simulink model "kyvadloMPC"  (R2018a)
settings: Solver=FixedStepAuto  StartTime=0.0  StopTime=10  FixedStep=Ts  MaxStep=0.01  RelTol=1e-3  EnableMultiTasking=on
PreLoadFcn:
  | m1=0.4;        % Hmotnost vozika [kg]
  | m2=0.08;      % Hmotnost kyvadla [kg]
  | l=0.2;            % Vzdialenost taziska od osi rotacie [m]
  | g=9.81;         % Tiazove zrychlenie [m/s2]
  | b=0.1;           % Koeficient trenia [m/s]
StartFcn:
  | kyvadloOfflineMPC
values from neighbouring files (symbols this model uses):
  Ac = -1/tau    (= -0.0166666666667)    [integrator.m]    (also in obmedzenia.m = [Acu;Acx]; stavovyprikaz.m = [-0.313 56.7 0; -0.0139 -0.426 0; 0 56.7 0]; testrozsirenieintegrator.m)
  b0 = [b0u; b0x]    [obmedzenia.m]
  B0 = [zeros(2*p5*nu,nx); B0x]    [obmedzenia.m]
  G = G+N((i-1)*nx+1:i*nx,:)'*P*M((i-1)*nx+1:i*nx,:)    [ucelovafunkcia.m]
  H = (H+H')/2    [.m]    (also in MPCuzavretaslucka.m; inkrementalny.m; integrator.m; kombinovaneobmedzenia.m)
  Ts = 5    [integrator.m]    (also in kyvadloOfflineLQ.m = kyvadlo.Ts; kyvadloOfflineMPC.m = kyvadlo.Ts; kyvadloOfflineMPCaKF.m = kyvadlo.Ts; stavovyprikaz.m = 0.5)
  uh = 0.002    [.m]    (also in MPCjedenkrok.m = 0.01; MPCuzavretaslucka.m = 0.01; integrator.m = 10; kombinovaneobmedzenia.m = 0.005)
  ul = -uh    (= -0.01)    [MPCjedenkrok.m]    (also in MPCuzavretaslucka.m; integrator.m = 0; kyvadloOfflineLQ.m = -5; kyvadloOfflineMPC.m = -5)
  x1h = 0.5    [kyvadloOfflineLQ.m]    (also in kyvadloOfflineMPC.m; kyvadloOfflineMPCaKF.m)
  x1l = -x1h    (= -0.5)    [kyvadloOfflineLQ.m]    (also in kyvadloOfflineMPC.m; kyvadloOfflineMPCaKF.m)
settings Model: Creator=UAMAI-LENOVO  LastModifiedBy=Gergely
settings DataIOCC: LimitDataPoints=on  SaveFormat=Array
settings OptimizationCC: LifeSpan=inf
settings DebuggingCC: SFUnexpectedBacktrackingDiag=warning  SFNoUnconditionalDefaultTransitionDiag=warning  SFExecutionAtInitializationDiag=none
settings HardwareCC: ProdBitPerPointer=32  ProdBitPerSizeT=32  ProdBitPerPtrDiffT=32  ProdLargestAtomicFloat=None  ProdIntDivRoundTo=Undefined  ProdEndianess=Unspecified  ProdWordSize=32  ProdHWDeviceType=32-bit Generic
settings ModelReferenceCC: PropagateSignalLabelsOutOfModel=off
settings CodeAppCC: StateflowObjectComments=on
settings GRTTargetCC: TargetLangStandard=C89/C90 (ANSI)  GeneratePreprocessorConditionals=Disable all
settings ConfigComp: CovMetricSettings=dw  CovHtmlReporting=on  CovSaveCumulativeToWorkspaceVar=on  CovSaveSingleToWorkspaceVar=on  CovExternalEMLEnable=off

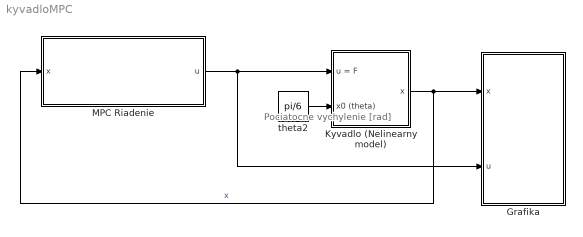
== system kyvadloMPC ==
  note: Pociatocne
      | vychylenie [rad]
  Grafika : Subsystem
  Kyvadlo (Nelinearny model) : Subsystem
  MPC Riadenie : Subsystem
  theta2 : Constant  Value=pi/6
  wires:
  theta2/1 -> Kyvadlo (Nelinearny model)/2(x0 (theta))
  Kyvadlo (Nelinearny model)/1(x) -> MPC Riadenie/1(x), Grafika/1(x)  "x"
  MPC Riadenie/1(u) -> Kyvadlo (Nelinearny model)/1(u = F), Grafika/2(u)

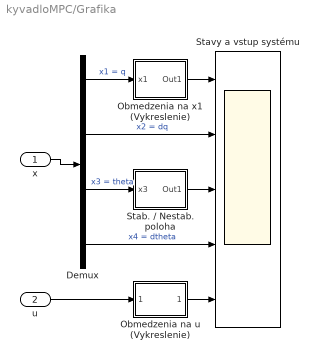
== system kyvadloMPC/Grafika ==
  x : Inport
  u : Inport  Port=2
  " Stavy a vstup systému" : Scope  NumInputPorts=5
  Demux : Demux
  Obmedzenia na u (Vykreslenie) : Subsystem
  "Obmedzenia na x1 (Vykreslenie) " : Subsystem
  Stab. / Nestab. poloha : Subsystem
  wires:
  Demux/2 -> " Stavy a vstup systému"/2  "x2 = dq"
  Demux/3 -> Stab. / Nestab. poloha/1(x3)  "x3 = theta"
  "Obmedzenia na x1 (Vykreslenie) "/1(Out1) -> " Stavy a vstup systému"/1
  u/1 -> Obmedzenia na u (Vykreslenie)/1(u = F)
  Demux/1 -> "Obmedzenia na x1 (Vykreslenie) "/1(x1)  "x1 = q"
  x/1 -> Demux/1
  Demux/4 -> " Stavy a vstup systému"/4  "x4 = dtheta"
  Stab. / Nestab. poloha/1(Out1) -> " Stavy a vstup systému"/3
  Obmedzenia na u (Vykreslenie)/1(Out1) -> " Stavy a vstup systému"/5

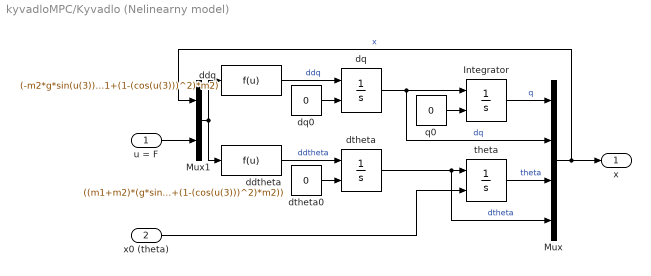
== system kyvadloMPC/Kyvadlo (Nelinearny model) ==
  u = F : Inport
  x0 (theta) : Inport  Port=2
  Integrator : Integrator  InitialConditionSource=external
  Mux : Mux
  Mux1 : Mux  Inputs=2
  ddq : Fcn  Expr=(-m2*g*sin(u(3))*cos(u(3))+m2*l*((u(4))^2)*sin(u(3))+b*m2*u(4)*cos(u(3))+u(5))/(m1+(1-(cos(u(3)))^2)*m2)
  ddtheta : Fcn  Expr=((m1+m2)*(g*sin(u(3))-b*u(4))-(m2*l*((u(4))^2)*sin(u(3))+u(5))*cos(u(3)))/(l*(m1+(1-(cos(u(3)))^2)*m2))
  dq : Integrator  InitialConditionSource=external
  dq0 : Constant  Value=0
  dtheta : Integrator  InitialConditionSource=external
  dtheta0 : Constant  Value=0
  q0 : Constant  Value=0
  theta : Integrator  InitialConditionSource=external
  x : Outport
  wires:
  Mux/1 -> x/1, Mux1/1  "x"
  ddq/1 -> dq/1  "ddq"
  dq/1 -> Mux/2, Integrator/1  "dq"
  ddtheta/1 -> dtheta/1  "ddtheta"
  x0 (theta)/1 -> theta/2
  q0/1 -> Integrator/2
  Integrator/1 -> Mux/1  "q"
  theta/1 -> Mux/3  "theta"
  dtheta/1 -> Mux/4, theta/1  "dtheta"
  Mux1/1 -> ddtheta/1, ddq/1
  dq0/1 -> dq/2
  dtheta0/1 -> dtheta/2
  u = F/1 -> Mux1/2

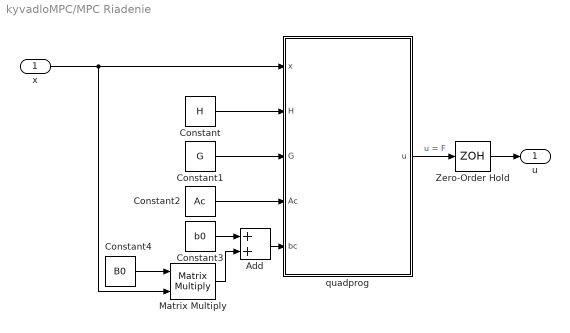
== system kyvadloMPC/MPC Riadenie ==
  x : Inport
  Add : Sum
  Constant : Constant  Value=H
  Constant1 : Constant  Value=G
  Constant2 : Constant  Value=Ac
  Constant3 : Constant  Value=b0
  Constant4 : Constant  Value=B0
  Matrix Multiply : Product  Multiplication=Matrix(*)
  Zero-Order Hold : ZeroOrderHold  SampleTime=Ts
  quadprog : MATLAB Function  InitFcn=kyvadloOfflineMPC  TreatAsAtomicUnit=on
  u : Outport
  wires:
  Matrix Multiply/1 -> Add/2
  Add/1 -> quadprog/5(bc)
  Constant3/1 -> Add/1
  Constant2/1 -> quadprog/4(Ac)
  Constant/1 -> quadprog/2(H)
  x/1 -> Matrix Multiply/2, quadprog/1(x)
  Constant1/1 -> quadprog/3(G)
  quadprog/1(u) -> Zero-Order Hold/1  "u = F"
  Constant4/1 -> Matrix Multiply/1
  Zero-Order Hold/1 -> u/1

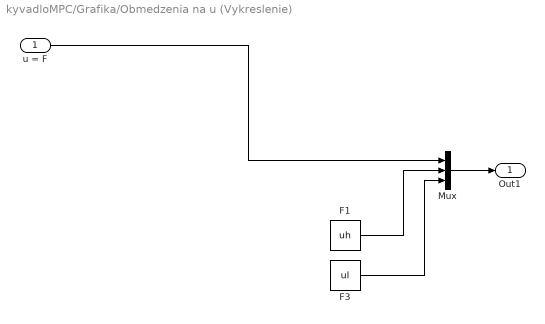
== system kyvadloMPC/Grafika/Obmedzenia na u (Vykreslenie) ==
  u = F : Inport
  F1 : Constant  Value=uh
  F3 : Constant  Value=ul
  Mux : Mux  Inputs=3
  Out1 : Outport
  wires:
  F1/1 -> Mux/2
  F3/1 -> Mux/3
  u = F/1 -> Mux/1
  Mux/1 -> Out1/1

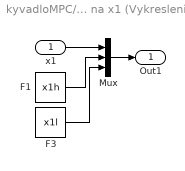
== system kyvadloMPC/Grafika/Obmedzenia na x1 (Vykreslenie)  ==
  x1 : Inport
  F1 : Constant  Value=x1h
  F3 : Constant  Value=x1l
  Mux : Mux  Inputs=3
  Out1 : Outport
  wires:
  F1/1 -> Mux/2
  F3/1 -> Mux/3
  x1/1 -> Mux/1
  Mux/1 -> Out1/1

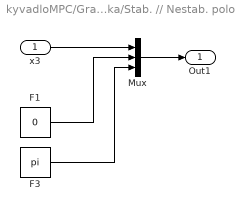
== system kyvadloMPC/Grafika/Stab. // Nestab. poloha ==
  x3 : Inport
  F1 : Constant  Value=0
  F3 : Constant  Value=pi
  Mux : Mux  Inputs=3
  Out1 : Outport
  wires:
  F1/1 -> Mux/2
  F3/1 -> Mux/3
  x3/1 -> Mux/1
  Mux/1 -> Out1/1

== matlab function kyvadloMPC/MPC Riadenie/quadprog ==
  data: x input; u output; H input; G input; Ac input; bc input
function u  = mpc(x,H,G,Ac,bc)
u=0; % Simulink output sizing
%Declare quadprog as extrinsic
coder.extrinsic('quadprog'); 
U=quadprog(H,G*x,Ac,bc);
u = U(1);
